simulink model "threeWayPercistentSwitch"  (R2017b)
settings: Solver=VariableStepAuto  StartTime=0.0  StopTime=10  RelTol=1e-3
libraries: simulink x2
settings Model: Creator=Niels Skov Vestergaa  LastModifiedBy=Niels Skov Vestergaa

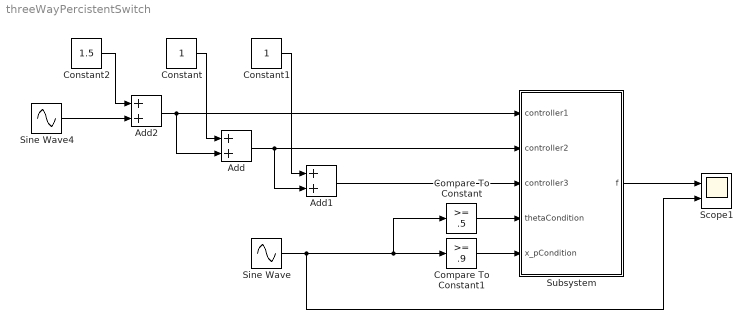
== system threeWayPercistentSwitch ==
  Add : Sum
  Add1 : Sum
  Add2 : Sum
  Compare To Constant : simulink/Logic and Bit Operations/Compare To Constant  relop=>=  const=.5  OutDataTypeStr=boolean
  Compare To Constant1 : simulink/Logic and Bit Operations/Compare To Constant  relop=>=  const=.9  OutDataTypeStr=boolean
  Constant : Constant
  Constant1 : Constant
  Constant2 : Constant  Value=1.5
  Scope1 : Scope  NumInputPorts=2
  Sine Wave : Sin  SampleTime=0
  Sine Wave4 : Sin  Amplitude=.1  Frequency=20  SampleTime=0
  Subsystem : Subsystem
  wires:
  Sine Wave/1 -> Scope1/2, Compare To Constant/1, Compare To Constant1/1
  Constant/1 -> Add/1
  Sine Wave4/1 -> Add2/2
  Add2/1 -> Add/2, Subsystem/1(controller1)
  Compare To Constant/1 -> Subsystem/4(thetaCondition)
  Compare To Constant1/1 -> Subsystem/5(x_pCondition)
  Subsystem/1(f) -> Scope1/1
  Constant2/1 -> Add2/1
  Add/1 -> Add1/2, Subsystem/2(controller2)
  Constant1/1 -> Add1/1
  Add1/1 -> Subsystem/3(controller3)

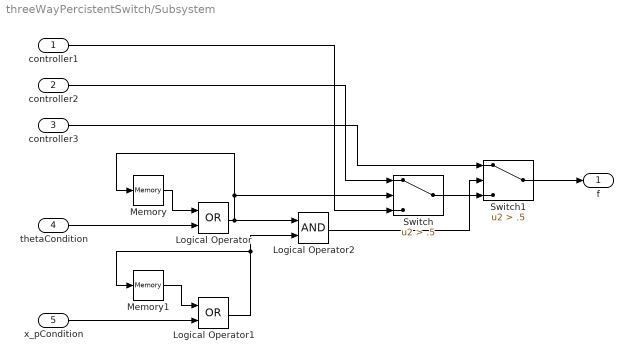
== system threeWayPercistentSwitch/Subsystem ==
  controller1 : Inport
  controller2 : Inport  Port=2
  controller3 : Inport  Port=3
  thetaCondition : Inport  Port=4
  x_pCondition : Inport  Port=5
  Logical Operator : Logic  Operator=OR  AllPortsSameDT=off  OutDataTypeStr=boolean
  Logical Operator1 : Logic  Operator=OR  AllPortsSameDT=off  OutDataTypeStr=boolean
  Logical Operator2 : Logic  AllPortsSameDT=off  OutDataTypeStr=boolean
  Memory : Memory
  Memory1 : Memory
  Switch : Switch  Criteria=u2 > Threshold  Threshold=.5
  Switch1 : Switch  Criteria=u2 > Threshold  Threshold=.5
  f : Outport
  wires:
  thetaCondition/1 -> Logical Operator/2
  Memory/1 -> Logical Operator/1
  Switch/1 -> Switch1/3
  controller3/1 -> Switch1/1
  controller1/1 -> Switch/3
  Memory1/1 -> Logical Operator1/1
  x_pCondition/1 -> Logical Operator1/2
  Logical Operator1/1 -> Logical Operator2/2, Memory1/1
  Switch1/1 -> f/1
  Logical Operator2/1 -> Switch1/2
  controller2/1 -> Switch/1
  Logical Operator/1 -> Memory/1, Switch/2, Logical Operator2/1
